simulink model "LibraryReference"
settings: Solver=FixedStepDiscrete  StartTime=0.0  StopTime=10.0  FixedStep=0.001
libraries: BusImpl x3, robot x1, robot2 x1, AtomicLibrary x1
settings SolverCC: AutoInsertRateTranBlk=on

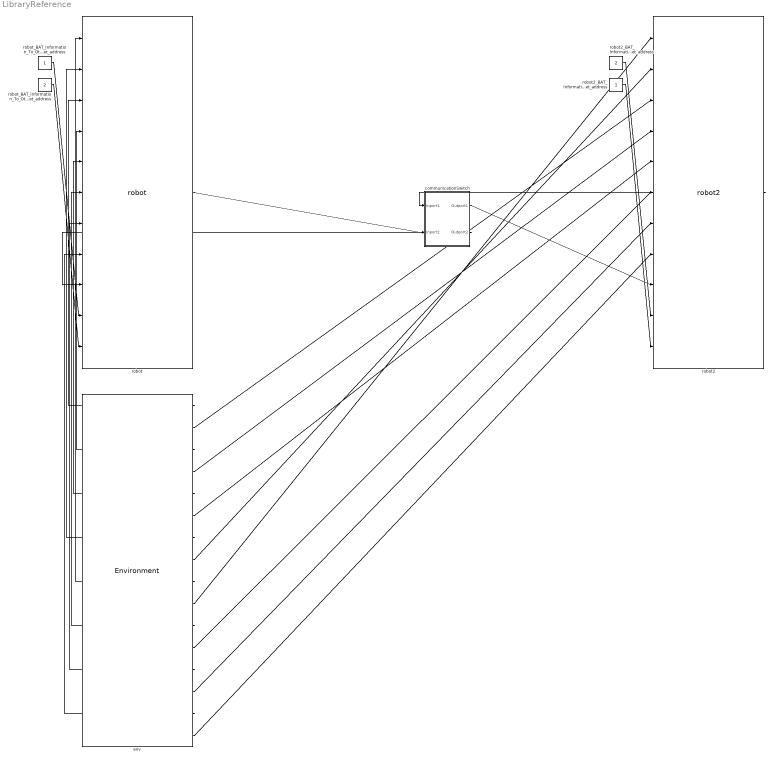
== system LibraryReference ==
  communicationSwitch : Subsystem  Tag=id=_FlgOAd8LEeKgPPszxxPBOg  LoadFcn=MainBusGenerator
  robot : robot/robot  Tag=id=_FlzI8N8LEeKgPPszxxPBOg
  robot2 : robot2/robot2  Tag=id=_Fl52oN8LEeKgPPszxxPBOg
  env : AtomicLibrary/Environment  Tag=id=_FmpdgN8LEeKgPPszxxPBOg
  robot_BAT_Information_To_OtherRobot_net_address : Constant  Tag=id=_F9cz8N8LEeKgPPszxxPBOg  Value=1  OutDataTypeMode=uint8  OutDataTypeStr=uint8
  robot2_BAT_Information_To_OtherRobot_net_address : Constant  Tag=id=_F9jhod8LEeKgPPszxxPBOg  Value=2  OutDataTypeMode=uint8  OutDataTypeStr=uint8
  robot2_BAT_Information_To_OtherRobot_send_receiver_net_address : Constant  Tag=id=_HBdOqd8LEeKgPPszxxPBOg  Value=1  OutDataTypeMode=uint8  OutDataTypeStr=uint8
  robot_BAT_Information_To_OtherRobot_send_receiver_net_address : Constant  Tag=id=_HBecwd8LEeKgPPszxxPBOg  Value=2  OutDataTypeMode=uint8  OutDataTypeStr=uint8
  wires:
  robot_BAT_Information_To_OtherRobot_net_address/1 -> robot/10
  robot2_BAT_Information_To_OtherRobot_net_address/1 -> robot2/10
  env/12 -> robot2/6
  env/2 -> robot2/3
  env/3 -> robot/4
  env/9 -> robot/1
  env/10 -> robot2/1
  env/5 -> robot/5
  env/6 -> robot2/5
  env/11 -> robot/6
  env/14 -> robot2/7
  env/8 -> robot2/2
  env/13 -> robot/7
  env/1 -> robot/3
  env/7 -> robot/2
  env/4 -> robot2/4
  env/16 -> robot2/8
  env/15 -> robot/8
  robot2/1 -> communicationSwitch/1(Inport1)
  robot/1 -> communicationSwitch/2(Inport2)
  communicationSwitch/2(Outport2) -> robot/9
  communicationSwitch/1(Outport1) -> robot2/9
  robot2_BAT_Information_To_OtherRobot_send_receiver_net_address/1 -> robot2/11
  robot_BAT_Information_To_OtherRobot_send_receiver_net_address/1 -> robot/11

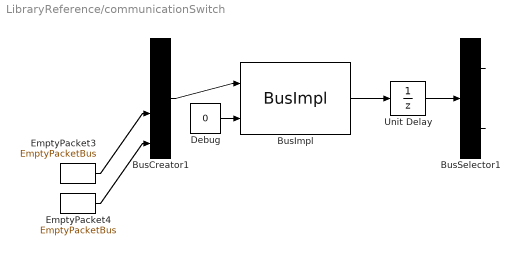
== system LibraryReference/communicationSwitch ==
  Inport1 : Inport  Tag=id=_HBdOpd8LEeKgPPszxxPBOg  Port=1  DataType=auto  OutDataType=fixdt(1, 16)  OutScaling=2^0  UseBusObject=on  OutDataTypeStr=Inherit: auto
      settings: BusObject=PacketBus
  Inport2 : Inport  Tag=id=_HBdOp98LEeKgPPszxxPBOg  Port=2  DataType=auto  OutDataType=fixdt(1, 16)  OutScaling=2^0  UseBusObject=on  OutDataTypeStr=Inherit: auto
      settings: BusObject=PacketBus
  Outport1 : Outport  Tag=id=_HBdOpt8LEeKgPPszxxPBOg  Port=1  DataType=auto  OutDataType=fixdt(1, 16)  OutScaling=2^0  UseBusObject=on  OutDataTypeStr=Inherit: auto
      settings: BusObject=PacketBus
  Outport2 : Outport  Tag=id=_HBdOqN8LEeKgPPszxxPBOg  Port=2  DataType=auto  OutDataType=fixdt(1, 16)  OutScaling=2^0  UseBusObject=on  OutDataTypeStr=Inherit: auto
      settings: BusObject=PacketBus
  BusCreator1 : BusCreator  Inputs=4  UseBusObject=on
      settings: BusObject=MainBus
  BusSelector1 : BusSelector  OutputSignals=rc1,rc2,rc3,rc4
  Unit Delay : UnitDelay  SampleTime=-1
  BusImpl : BusImpl/BusImpl
  Debug : Constant  Value=0  OutDataType=fixdt(1, 16)  OutScaling=2^0
  EmptyPacket3 : BusImpl/EmptyPacketBus
  EmptyPacket4 : BusImpl/EmptyPacketBus
  wires:
  BusImpl/1 -> Unit Delay/1
  BusCreator1/1 -> BusImpl/1
  Unit Delay/1 -> BusSelector1/1
  Inport1/1 -> BusCreator1/1  "rc1"
  Inport2/1 -> BusCreator1/2  "rc2"
  BusSelector1/1 -> Outport1/1
  BusSelector1/2 -> Outport2/1
  Debug/1 -> BusImpl/2
  EmptyPacket3/1 -> BusCreator1/3
  EmptyPacket4/1 -> BusCreator1/4
